simulink model "pi_sat"  (R2017a)
settings: Solver=ode45  StartTime=0.0  StopTime=30  RelTol=1e-3  EnableMultiTasking=on
values from neighbouring files (symbols this model uses):
  Ki = vals(2)    [bbbc.m]    (also in geneticalgortihm.m = x(2); optimal.m = x(2))
  Kp = vals(1)    [bbbc.m]    (also in geneticalgortihm.m = x(1); optimal.m = x(1))
settings Model: Creator=Benay  LastModifiedBy=musti
settings DataIOCC: LimitDataPoints=on  SaveFormat=Array
settings OptimizationCC: LifeSpan=inf
settings DebuggingCC: SFUnexpectedBacktrackingDiag=warning  SFNoUnconditionalDefaultTransitionDiag=warning  SFExecutionAtInitializationDiag=none
settings HardwareCC: ProdBitPerPointer=32  ProdBitPerSizeT=32  ProdBitPerPtrDiffT=32  ProdLargestAtomicFloat=None  ProdIntDivRoundTo=Undefined  ProdEndianess=Unspecified  ProdWordSize=32  ProdHWDeviceType=32-bit Generic
settings ModelReferenceCC: PropagateSignalLabelsOutOfModel=off
settings GRTTargetCC: TargetLangStandard=C89/C90 (ANSI)  GeneratePreprocessorConditionals=Disable all
settings ConfigComp: CovMetricSettings=dw  CovHtmlReporting=on  CovSaveCumulativeToWorkspaceVar=on  CovSaveSingleToWorkspaceVar=on  CovExternalEMLEnable=off

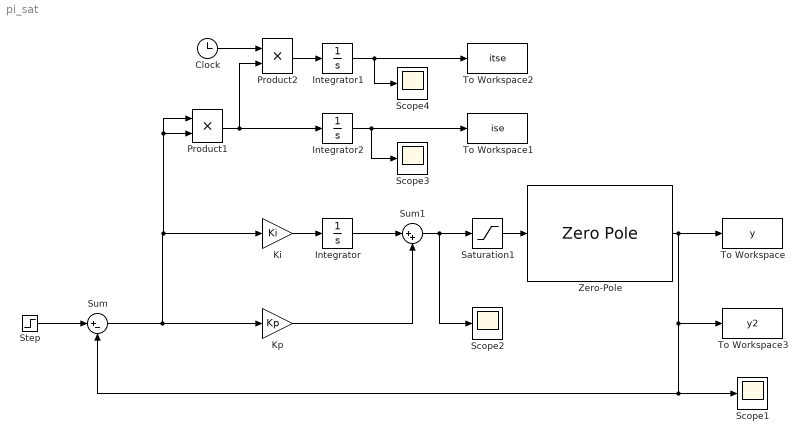
== system pi_sat ==
  Clock : Clock
  Integrator : Integrator
  Integrator1 : Integrator
  Integrator2 : Integrator
  Ki : Gain  Gain=Ki
  Kp : Gain  Gain=Kp
  Product1 : Product
  Product2 : Product
  Saturation1 : Saturate  UpperLimit=10  LowerLimit=-10  LinearizeAsGain=off  ZeroCross=off
  Scope{1..4} (4 alike) : Scope
  Step : Step  Time=0  SampleTime=0
  Sum : Sum  Inputs=|+-
  Sum1 : Sum  Inputs=|++
  To Workspace : ToWorkspace  VariableName=y  SampleTime=-1
      settings: Save2DSignal=2-D array (concatenate along first dimension)
  To Workspace1 : ToWorkspace  VariableName=ise  SampleTime=-1
  To Workspace2 : ToWorkspace  VariableName=itse  SampleTime=-1
  To Workspace3 : ToWorkspace  VariableName=y2  SaveFormat=Structure With Time  SampleTime=-1
      settings: Save2DSignal=2-D array (concatenate along first dimension)
  Zero-Pole : ZeroPole  Zeros=[-7.5]  Poles=[2i -2i]  Gain=[10]
  wires:
  Step/1 -> Sum/1
  Sum/1 -> Ki/1, Product1/1, Product1/2, Kp/1
  Kp/1 -> Sum1/2
  Product1/1 -> Product2/2, Integrator2/1
  Integrator2/1 -> Scope3/1, To Workspace1/1
  Ki/1 -> Integrator/1
  Integrator/1 -> Sum1/1
  Product2/1 -> Integrator1/1
  Integrator1/1 -> Scope4/1, To Workspace2/1
  Zero-Pole/1 -> Scope1/1, Sum/2, To Workspace3/1, To Workspace/1
  Sum1/1 -> Saturation1/1, Scope2/1
  Clock/1 -> Product2/1
  Saturation1/1 -> Zero-Pole/1
